simulink model "RobustMPCInput_mdl"  (R2013a)
settings: Solver=ode45  StartTime=0.0  StopTime=10.0  RelTol=1e-3
undefined symbols (not defined in the file): TTR_RobustMPC
settings Model: Creator=Kostas  LastModifiedBy=Kostas

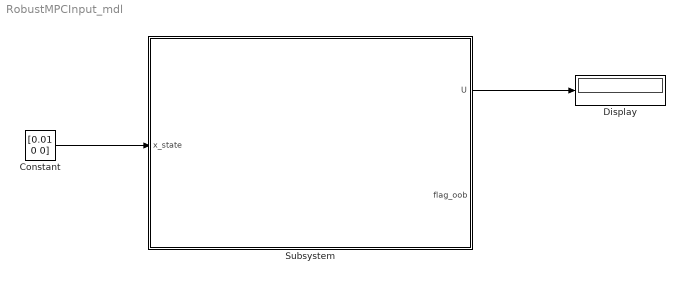
== system RobustMPCInput_mdl ==
  Constant : Constant  Value=[0.01 0 0]
  Display : Display
  Subsystem : Subsystem  mask{H=TTR_RobustMPC.Zdir.Explicit.H, K=TTR_RobustMPC.Zdir.Explicit.K, F=TTR_RobustMPC.Zdir.Explicit.F, G=TTR_RobustMPC.Zdir.Explicit.G, Nc=TTR_RobustMPC.Zdir.Explicit.Nc, Nx=TTR_RobustMPC.Zdir.Explicit.Nx, Hi_init=zeros(100,TTR_RobustMPC.Zdir.Explicit.Nx)}
      mask prompts: H "Explicit Robust MPC {H}"; K "Explicit Robust MPC {K}"; F "Explicit Robust MPC {F}"; G "Explicit Robust MPC {G}"; Nc "Explicit Robust MPC {Nc}"; Nx "Explicit Robust MPC {Nx}"; Hi_init "Explicit Robust MPC {Hinit}"
      mask Display:
      | port_label('input',1,'x_state');
      | port_label('output',1,'U');
      | port_label('output',2,'flag_oob');
      | disp('Explicit Robust MPC')
      | plot([10 20 30 40],[10 20 20 25])
  wires:
  Constant/1 -> Subsystem/1(x_state)
  Subsystem/1(U) -> Display/1

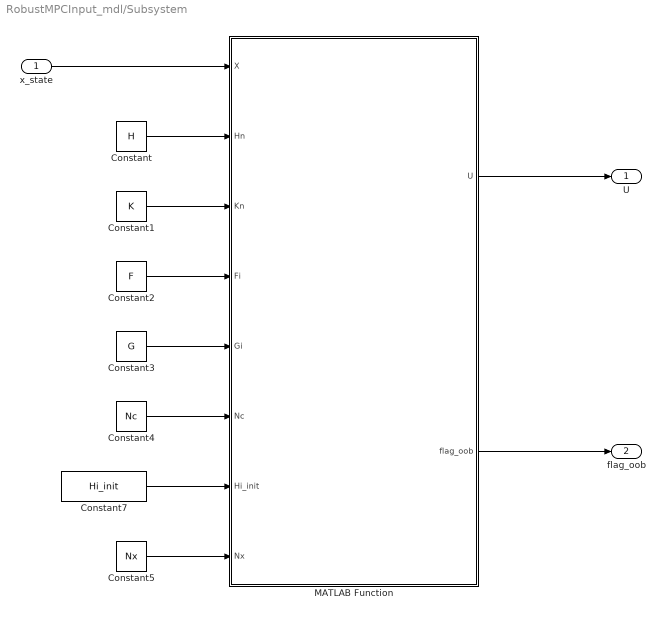
== system RobustMPCInput_mdl/Subsystem ==
  x_state : Inport
  Constant : Constant  Value=H
  Constant1 : Constant  Value=K
  Constant2 : Constant  Value=F
  Constant3 : Constant  Value=G
  Constant4 : Constant  Value=Nc
  Constant5 : Constant  Value=Nx
  Constant7 : Constant  Value=Hi_init
  MATLAB Function : MATLAB Function  TreatAsAtomicUnit=on
  U : Outport
  flag_oob : Outport  Port=2
  wires:
  Constant/1 -> MATLAB Function/2(Hn)
  Constant1/1 -> MATLAB Function/3(Kn)
  Constant2/1 -> MATLAB Function/4(Fi)
  Constant3/1 -> MATLAB Function/5(Gi)
  Constant4/1 -> MATLAB Function/6(Nc)
  Constant5/1 -> MATLAB Function/8(Nx)
  Constant7/1 -> MATLAB Function/7(Hi_init)
  x_state/1 -> MATLAB Function/1(X)
  MATLAB Function/1(U) -> U/1
  MATLAB Function/2(flag_oob) -> flag_oob/1

== matlab function RobustMPCInput_mdl/Subsystem/MATLAB Function ==
  data: X input; U output; Hn input; Kn input; Fi input; Gi input; Nc input; Hi_init input; Nx input; flag_oob output
function[U,flag_oob] = OptimalMPCInput_mdl(X,Hn,Kn,Fi,Gi,Nc,Hi_init,Nx)
%#codegen

tolerance = 1;
nr  = size(Nc,1);
MPT_ABSTOL = 1e-8;
minreg = 0;
X = round(10000*X)/10000;

flag_oob = 0;
%maxSize = max(Nc);

%Hi = zeros(100,3);
Hi = Hi_init;

Ki = zeros(1000,1);

% Find the proper region
abspos = 1;
for ireg = 1:nr
    sumViol = 0;
    isinside = 1;
    

  %  Hi(1:Nc(ireg),1:4) = Hn(abspos:(abspos+Nc(ireg)-1),1:4);
    for i = 1:Nc(ireg)
        for j = 1:Nx
            Hi(i,j) = Hn(abspos + i - 1,j);
        end
    end
    
%    Ki(1:Nc(ireg),1) = Kn(abspos:(abspos+Nc(ireg)-1),1);
    for i = 1:Nc(ireg)
        Ki(i,1) = Kn(abspos + i - 1,1);
    end
    abspos = abspos + Nc(ireg);
    
    F = Fi(ireg,:);
    G = Gi(ireg,:);
    
    nc = Nc(ireg);
    
    for ic = 1:nc
        hx = Hi(ic,:)*X;
        if ((hx - Ki(ic)) > MPT_ABSTOL)
            isinside = 0;
            sumViol = sumViol + (hx - Ki(ic));
        end
    end
    
    if (sumViol < tolerance)
        tolerance = sumViol;
        minreg = ireg;
    end
    % extract the right control law
    if (isinside == 1)
        U = F*X + G;
        return
    end
end
F = Fi(minreg,:);
G = Gi(minreg,:);
U = F*X + G;
flag_oob = 1;
return
